simulink model "Ex_2_10_solver"  (R2020b)
settings: Solver=VariableStepAuto  StartTime=0.0  StopTime=10.0  RelTol=1e-3
values from neighbouring files (symbols this model uses):
  damping = 0    [Ex2.m]    (also in Ex2_9.m; Ex_2_10.m)
  mass = 750    [Ex1.m]    (also in Ex2.m; Ex2_9.m; Ex4.m = 1000; Ex5.m = 1000)
  stiffness = 50000    [Ex1.m]    (also in Ex2.m; Ex2_9.m; Ex_2_10.m)
  x_0 = 0.01    [Ex1.m]    (also in Ex2.m; Ex2_9.m; Ex4.m = 0.1; Ex5.m = 0.1)
  x_dot_0 = 0.2    [Ex1.m]    (also in Ex2.m = 0; Ex2_9.m = 0; Ex4.m = 0; Ex5.m = 0)
settings Model: Creator=Ricardo Fitas  LastModifiedBy=Ricardo Fitas

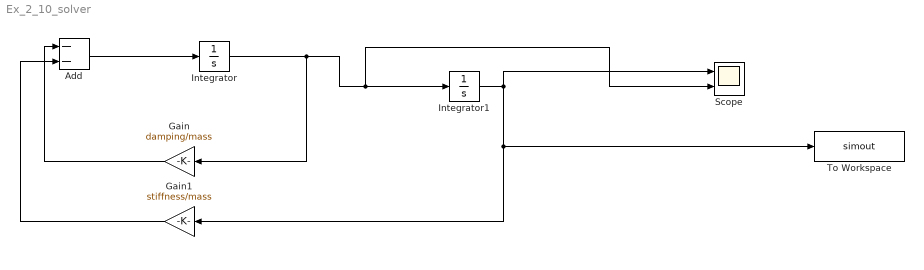
== system Ex_2_10_solver ==
  Add : Sum  Inputs=--
  Gain : Gain  Gain=damping/mass
  Gain1 : Gain  Gain=stiffness/mass
  Integrator : Integrator  InitialCondition=x_0
  Integrator1 : Integrator  InitialCondition=x_dot_0
  Scope : Scope  NumInputPorts=2
  To Workspace : ToWorkspace  VariableName=simout  SaveFormat=Timeseries  SampleTime=-1
  wires:
  Add/1 -> Integrator/1
  Gain/1 -> Add/1
  Gain1/1 -> Add/2
  Integrator1/1 -> To Workspace/1, Gain1/1, Scope/1
  Integrator/1 -> Gain/1, Scope/2, Integrator1/1
